simulink model "esempio1_farrell"  (R2025b)
settings: Solver=ode45  StartTime=0.0  StopTime=100  RelTol=1e-3  EnableMultiTasking=on
libraries: simulink x1
settings Model: Creator=C.Perri  LastModifiedBy=Steph
settings SolverCC: AlgebraicLoopSolver=TrustRegion
settings DataIOCC: LimitDataPoints=on  SaveFormat=Array  SignalLoggingSaveFormat=ModelDataLogs  ReturnWorkspaceOutputs=off
settings OptimizationCC: InitFltsAndDblsToZero=on  LifeSpan=inf
settings DebuggingCC: SaveWithParameterizedLinksMsg=none  UnderspecifiedInitializationDetection=Classic  MergeDetectMultiDrivingBlocksExec=none  SignalResolutionControl=TryResolveAllWithWarning  SolverPrmCheckMsg=warning  MultiTaskDSMMsg=warning  MultiTaskCondExecSysMsg=none  FcnCallInpInsideContextMsg=warning  UnconnectedInputMsg=warning  UnconnectedOutputMsg=warning  UnconnectedLineMsg=warning  SFUnexpectedBacktrackingDiag=warning  SFNoUnconditionalDefaultTransitionDiag=warning  SFExecutionAtInitializationDiag=none  ArithmeticOperatorsInVariantConditions=warning
settings HardwareCC: ProdBitPerPointer=32.0  ProdBitPerSizeT=32.0  ProdBitPerPtrDiffT=32.0  ProdLargestAtomicFloat=None  ProdIntDivRoundTo=Undefined  ProdEndianess=Unspecified  ProdWordSize=32.0  ProdHWDeviceType=32-bit Generic
settings ModelReferenceCC: EnableRefExpFcnMdlSchedulingChecks=on  PropagateSignalLabelsOutOfModel=off
settings RTWCC: GPUComputeCapability=3.5
settings CodeAppCC: StateflowObjectComments=on
settings GRTTargetCC: TargetFcnLib=ansi_tfl_tmw.mat  TargetLangStandard=C89/C90 (ANSI)  CombineOutputUpdateFcns=off  GRTInterface=on
settings ConfigComp: CovMetricSettings=dw  CovSaveCumulativeToWorkspaceVar=on  CovSaveSingleToWorkspaceVar=on

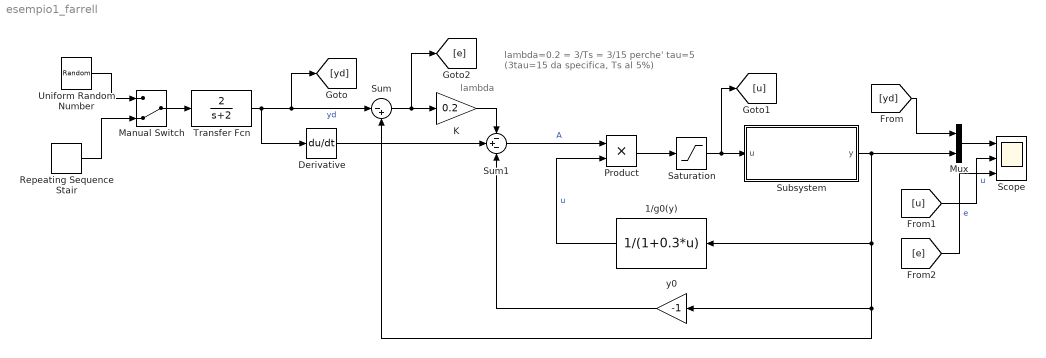
== system esempio1_farrell ==
  note: lambda
  note: lambda=0.2 = 3/Ts = 3/15
      |  perche' tau=5 (3tau=15 da specifica, Ts al 5%)
  1/g0(y) : Fcn  Expr=1/(1+0.3*u)
  Derivative : Derivative
  K : Gain  Gain=0.2
  Manual Switch : ManualSwitch  CurrentSetting=0
  Mux : Mux  Inputs=2
  Product : Product  RndMeth=Zero
  Repeating Sequence Stair : simulink/Sources/Repeating Sequence Stair  OutValues=[20 60].'  tsamp=10  OutMin=[]  OutMax=[]  OutDataTypeStr=float('double')  OutputDataTypeScalingMode=Specify via dialog  OutDataType=float('double')  ConRadixGroup=Best Precision: Vector-wise  OutScaling=2^-12
  Saturation : Saturate  UpperLimit=10  LowerLimit=-10
  Scope : Scope  NumInputPorts=3
      settings: TimeSpan=100  ActiveDisplayYMinimum=-13.0265353382887  ActiveDisplayYMaximum=117.23881804459833
  Subsystem : Subsystem
  Sum : Sum  Inputs=|-+
  Sum1 : Sum  Inputs=-+-
  Transfer Fcn : TransferFcn  Numerator=[2]  Denominator=[1 2]
  Uniform Random Number : UniformRandomNumber  Minimum=20  Maximum=60  SampleTime=10
  y0 : Gain  Gain=-1
  wires:
  Subsystem/1(y) -> Mux/2, y0/1, Sum/2, 1/g0(y)/1
  Transfer Fcn/1 -> Derivative/1, Sum/1, [yd]  "yd"
  y0/1 -> Sum1/3
  Sum/1 -> [e], K/1
  K/1 -> Sum1/1
  Derivative/1 -> Sum1/2
  [yd] -> Mux/1
  Mux/1 -> Scope/1
  1/g0(y)/1 -> Product/2  "u"
  Product/1 -> Saturation/1
  Manual Switch/1 -> Transfer Fcn/1
  Uniform Random Number/1 -> Manual Switch/1
  Repeating Sequence Stair/1 -> Manual Switch/2
  Saturation/1 -> Subsystem/1(u), [u]
  [u] -> Scope/2  "u"
  Sum1/1 -> Product/1  "A"
  [e] -> Scope/3  "e"

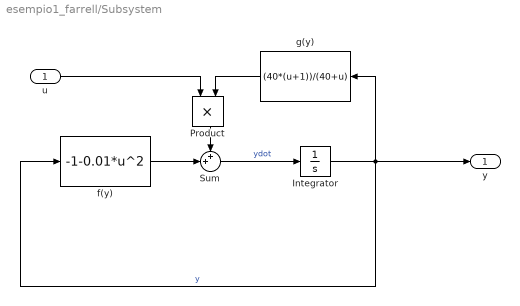
== system esempio1_farrell/Subsystem ==
  u : Inport
  Integrator : Integrator
  Product : Product  RndMeth=Zero
  Sum : Sum  Inputs=++|
  f(y) : Fcn  Expr=-1-0.01*u^2
  g(y) : Fcn  Expr=(40*(u+1))/(40+u)
  y : Outport
  wires:
  Sum/1 -> Integrator/1  "ydot"
  f(y)/1 -> Sum/2
  Product/1 -> Sum/1
  g(y)/1 -> Product/2
  u/1 -> Product/1
  Integrator/1 -> y/1, g(y)/1, f(y)/1  "y"
